simulink model "dong_hoc_thuan"  (R2018b)
settings: Solver=VariableStepAuto  StartTime=0.0  StopTime=10.0  RelTol=1e-3  EnableMultiTasking=on
settings Model: Creator=admin  LastModifiedBy=khina
settings OptimizationCC: LifeSpan=inf
settings DebuggingCC: SFUnexpectedBacktrackingDiag=warning  SFNoUnconditionalDefaultTransitionDiag=warning
settings SFSimCC: SimUseLocalCustomCode=off
settings RTWCC: RTWUseLocalCustomCode=off
settings CodeAppCC: StateflowObjectComments=on
settings GRTTargetCC: TargetLangStandard=C89/C90 (ANSI)  GeneratePreprocessorConditionals=Disable all
settings ConfigComp: CovMetricSettings=dw  CovHtmlReporting=on  CovSaveCumulativeToWorkspaceVar=on  CovSaveSingleToWorkspaceVar=on  CovExternalEMLEnable=off

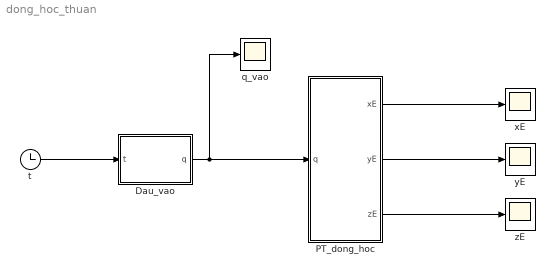
== system dong_hoc_thuan ==
  Dau_vao : MATLAB Function  TreatAsAtomicUnit=on
  PT_dong_hoc : MATLAB Function  TreatAsAtomicUnit=on
  q_vao : Scope
  "t " : Clock
  xE : Scope
  yE : Scope
  zE : Scope
  wires:
  "t "/1 -> Dau_vao/1(t)
  Dau_vao/1(q) -> q_vao/1, PT_dong_hoc/1(q)
  PT_dong_hoc/1(xE) -> xE/1
  PT_dong_hoc/2(yE) -> yE/1
  PT_dong_hoc/3(zE) -> zE/1

== matlab function dong_hoc_thuan/PT_dong_hoc ==
  data: q input; xE output; yE output; zE output
function [xE,yE,zE] = fcn(q)
d1=0.3;
d2=0.3;
d3=0.2;
d4=0.1;
d5=0.08;
d6 = 0.08;
%PT diem cuoi xE,yE,zE
xE = -cos(q(1,1)) * cos(q(2,1)) * sin(q(5,1)) * sin(q(3,1)) * sin(q(4,1)) * d6 + cos(q(1,1)) * cos(q(2,1)) * sin(q(5,1)) * cos(q(4,1)) * cos(q(3,1)) * d6 + cos(q(1,1)) * cos(q(2,1)) * cos(q(5,1)) * sin(q(3,1)) * cos(q(4,1)) * d6 + cos(q(1,1)) * cos(q(2,1)) * cos(q(5,1)) * cos(q(3,1)) * sin(q(4,1)) * d6 + sin(q(1,1)) * sin(q(2,1)) * sin(q(5,1)) * sin(q(3,1)) * sin(q(4,1)) * d6 - sin(q(1,1)) * sin(q(2,1)) * sin(q(5,1)) * cos(q(4,1)) * cos(q(3,1)) * d6 - sin(q(1,1)) * sin(q(2,1)) * cos(q(5,1)) * sin(q(3,1)) * cos(q(4,1)) * d6 - sin(q(1,1)) * sin(q(2,1)) * cos(q(5,1)) * cos(q(3,1)) * sin(q(4,1)) * d6 - cos(q(1,1)) * cos(q(2,1)) * sin(q(3,1)) * sin(q(4,1)) * d3 + cos(q(1,1)) * cos(q(2,1)) * cos(q(4,1)) * cos(q(3,1)) * d3 + sin(q(1,1)) * sin(q(2,1)) * sin(q(3,1)) * sin(q(4,1)) * d3 - sin(q(1,1)) * sin(q(2,1)) * cos(q(4,1)) * cos(q(3,1)) * d3 + cos(q(1,1)) * cos(q(2,1)) * cos(q(3,1)) * d2 - sin(q(1,1)) * sin(q(2,1)) * cos(q(3,1)) * d2 + cos(q(1,1)) * sin(q(2,1)) * d4 + cos(q(1,1)) * sin(q(2,1)) * d5 + cos(q(2,1)) * sin(q(1,1)) * d4 + cos(q(2,1)) * sin(q(1,1)) * d5;
yE = -cos(q(1,1)) * sin(q(2,1)) * sin(q(5,1)) * sin(q(3,1)) * sin(q(4,1)) * d6 + cos(q(1,1)) * sin(q(2,1)) * sin(q(5,1)) * cos(q(4,1)) * cos(q(3,1)) * d6 + cos(q(1,1)) * sin(q(2,1)) * cos(q(5,1)) * sin(q(3,1)) * cos(q(4,1)) * d6 + cos(q(1,1)) * sin(q(2,1)) * cos(q(5,1)) * cos(q(3,1)) * sin(q(4,1)) * d6 - cos(q(2,1)) * sin(q(1,1)) * sin(q(5,1)) * sin(q(3,1)) * sin(q(4,1)) * d6 + cos(q(2,1)) * sin(q(1,1)) * sin(q(5,1)) * cos(q(4,1)) * cos(q(3,1)) * d6 + cos(q(2,1)) * sin(q(1,1)) * cos(q(5,1)) * sin(q(3,1)) * cos(q(4,1)) * d6 + cos(q(2,1)) * sin(q(1,1)) * cos(q(5,1)) * cos(q(3,1)) * sin(q(4,1)) * d6 - cos(q(1,1)) * sin(q(2,1)) * sin(q(3,1)) * sin(q(4,1)) * d3 + cos(q(1,1)) * sin(q(2,1)) * cos(q(3,1)) * cos(q(4,1)) * d3 - cos(q(2,1)) * sin(q(1,1)) * sin(q(3,1)) * sin(q(4,1)) * d3 + cos(q(2,1)) * sin(q(1,1)) * cos(q(3,1)) * cos(q(4,1)) * d3 + cos(q(1,1)) * sin(q(2,1)) * cos(q(3,1)) * d2 + cos(q(2,1)) * sin(q(1,1)) * cos(q(3,1)) * d2 - cos(q(1,1)) * cos(q(2,1)) * d4 - cos(q(1,1)) * cos(q(2,1)) * d5 + sin(q(1,1)) * sin(q(2,1)) * d4 + sin(q(1,1)) * sin(q(2,1)) * d5;
zE = sin(q(5,1)) * sin(q(3,1)) * cos(q(4,1)) * d6 + sin(q(5,1)) * cos(q(3,1)) * sin(q(4,1)) * d6 + cos(q(5,1)) * sin(q(3,1)) * sin(q(4,1)) * d6 - cos(q(5,1)) * cos(q(4,1)) * cos(q(3,1)) * d6 + sin(q(3,1)) * d3 * cos(q(4,1)) + cos(q(3,1)) * d3 * sin(q(4,1)) + d2 * sin(q(3,1)) + d1;
end

== matlab function dong_hoc_thuan/Dau_vao ==
  data: t input; q output
function q = fcn(t)
%dau vao khai bao cac bien khop
q=zeros(6,1);
q(1,1)=sin(t+pi/3);
q(2,1)=sin(t);
q(3,1)=cos(t);
q(4,1)=sin((pi/2)*t);
q(5,1)=cos(t);
q(6,1)= cos(t + pi/4);
end
